simulink model "series_link_blance_leg"  (R2022b)
settings: Solver=ode45  StartTime=0.0  StopTime=14  MaxStep=0.2  RelTol=1e-3
values from neighbouring files (symbols this model uses):
  a11 = polyfit(leg,k11,2)    [series_get_k.m]
  a12 = polyfit(leg,k12,2)    [series_get_k.m]
  a13 = polyfit(leg,k13,1)    [series_get_k.m]
  a14 = polyfit(leg,k14,2)    [series_get_k.m]
  N = mp*diff(x + L*sin(theta),t,2)    [series_get_k1_length.m]
undefined symbols (not defined in the file or in its folder): X, Y, Z
libraries: sm_lib x74, nesl_utility x17, slpidlib x2, cstblocks x2, matrix_library x2
(part 3 of 3)

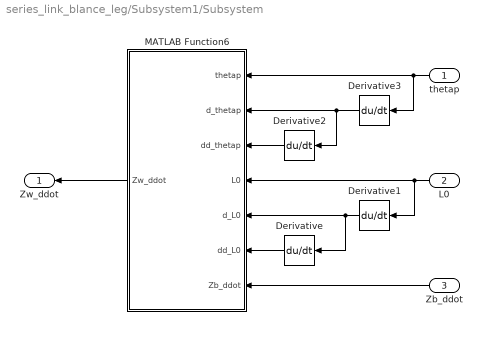
== system series_link_blance_leg/Subsystem1/Subsystem ==
  thetap : Inport
  L0 : Inport  Port=2
  Zb_ddot : Inport  Port=3
  Derivative{,1..3} (4 alike) : Derivative
  MATLAB Function6 : MATLAB Function  TreatAsAtomicUnit=on
  Zw_ddot : Outport
  wires:
  thetap/1 -> MATLAB Function6/1(thetap), Derivative3/1
  L0/1 -> Derivative1/1, MATLAB Function6/4(L0)
  Derivative1/1 -> Derivative/1, MATLAB Function6/5(d_L0)
  Derivative2/1 -> MATLAB Function6/3(dd_thetap)
  Derivative3/1 -> Derivative2/1, MATLAB Function6/2(d_thetap)
  Derivative/1 -> MATLAB Function6/6(dd_L0)
  Zb_ddot/1 -> MATLAB Function6/7(Zb_ddot)
  MATLAB Function6/1(Zw_ddot) -> Zw_ddot/1

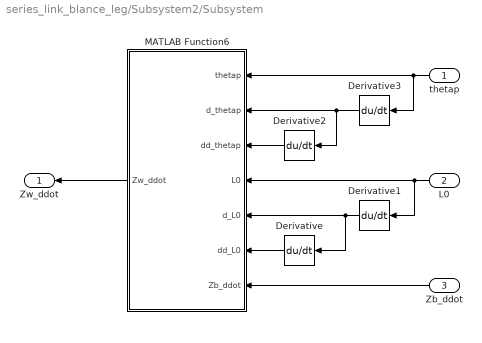
== system series_link_blance_leg/Subsystem2/Subsystem ==
  thetap : Inport
  L0 : Inport  Port=2
  Zb_ddot : Inport  Port=3
  Derivative{,1..3} (4 alike) : Derivative
  MATLAB Function6 : MATLAB Function  TreatAsAtomicUnit=on
  Zw_ddot : Outport
  wires:
  MATLAB Function6/1(Zw_ddot) -> Zw_ddot/1
  Zb_ddot/1 -> MATLAB Function6/7(Zb_ddot)
  Derivative/1 -> MATLAB Function6/6(dd_L0)
  Derivative3/1 -> MATLAB Function6/2(d_thetap), Derivative2/1
  Derivative2/1 -> MATLAB Function6/3(dd_thetap)
  Derivative1/1 -> MATLAB Function6/5(d_L0), Derivative/1
  L0/1 -> MATLAB Function6/4(L0), Derivative1/1
  thetap/1 -> Derivative3/1, MATLAB Function6/1(thetap)

== matlab function series_link_blance_leg/calc1/MATLAB Function6 ==
  data: k output; a input; length input
function k = get_K(a,length)
   k = polyval(a,length);  
end

== matlab function series_link_blance_leg/Subsystem1/Subsystem/MATLAB Function6 ==
  data: thetap input; Zw_ddot output; d_thetap input; dd_thetap input; L0 input; d_L0 input; dd_L0 input; Zb_ddot input
function Zw_ddot = Zw_ddot_calc(thetap,d_thetap,dd_thetap,L0,d_L0,dd_L0,Zb_ddot)

   Zw_ddot=Zb_ddot-dd_L0*cos(thetap)+2*d_L0*d_thetap*sin(thetap)+L0*dd_thetap*sin(thetap)+L0*(d_thetap^2)*cos(thetap);
end

== matlab function series_link_blance_leg/Subsystem1/MATLAB Function6 ==
  data: thetap input; zw_ddot input; F input; Fn output
function Fn = Fn_calc(thetap,zw_ddot,F)
    
  Mp=5.54; 
  Mw=1.18;
  g=9.8;
  Fn=F*cos(thetap)+Mp*g+Mw*zw_ddot;
end

== matlab function series_link_blance_leg/Subsystem2/MATLAB Function6 ==
  data: thetap input; zw_ddot input; F input; Fn output
function Fn = Fn_calc(thetap,zw_ddot,F)
    
  Mp=5.54; 
  Mw=1.18;
  g=9.8;
  Fn=F*cos(thetap)+Mp*g+Mw*zw_ddot;
end

== matlab function series_link_blance_leg/Subsystem2/Subsystem/MATLAB Function6 ==
  data: thetap input; Zw_ddot output; d_thetap input; dd_thetap input; L0 input; d_L0 input; dd_L0 input; Zb_ddot input
function Zw_ddot = Zw_ddot_calc(thetap,d_thetap,dd_thetap,L0,d_L0,dd_L0,Zb_ddot)

   Zw_ddot=Zb_ddot-dd_L0*cos(thetap)+2*d_L0*d_thetap*sin(thetap)+L0*dd_thetap*sin(thetap)+L0*(d_thetap^2)*cos(thetap);
end

== matlab function series_link_blance_leg/control1/MATLAB Function6 ==
  data: F0 input; T_joint output; theta1 input
function T_joint = VMC_calc(F0,theta1)
    l1 = 0.163; %%163.04mm
    l2 = 0.165; %%164.75mm
    l3 = 0.170; %%170.15mm
    l4 = 0.08;  %%79.5mm
    l23 = 0.04;  %%40.05mm

    J = l2*cos(theta1) + l1*cos(theta1 + acos((l2^2 - 2*cos(pi/4 + theta1)*l2*l4 - l3^2 + l4^2 + l23^2)/(2*l23*(l2^2 - 2*cos(pi/4 + theta1)*l2*l4 + l4^2)^(1/2))) + asin((l4*sin(theta1 + pi/4))/(l2^2 - 2*cos(pi/4 + theta1)*l2*l4 + l4^2)^(1/2)))*(((l4*cos(theta1 + pi/4))/(l2^2 - 2*cos(pi/4 + theta1)*l2*l4 + l4^2)^(1/2) - (l2*l4^2*sin(theta1 + pi/4)^2)/(l2^2 - 2*cos(pi/4 + theta1)*l2*l4 + l4^2)^(3/2))/(1 - (l4^2*sin(theta1 + pi/4)^2)/(l2^2 - 2*cos(pi/4 + theta1)*l2*l4 + l4^2))^(1/2) - ((l2*l4*sin(theta1 + pi/4))/(l23*(l2^2 - 2*cos(pi/4 + theta1)*l2*l4 + l4^2)^(1/2)) - (l2*l4*sin(theta1 + pi/4)*(l2^2 - 2*cos(pi/4 + theta1)*l2*l4 - l3^2 + l4^2 + l23^2))/(2*l23*(l2^2 - 2*cos(pi/4 + theta1)*l2*l4 + l4^2)^(3/2)))/(1 - (l2^2 - 2*cos(pi/4 + theta1)*l2*l4 - l3^2 + l4^2 + l23^2)^2/(4*l23^2*(l2^2 - 2*cos(pi/4 + theta1)*l2*l4 + l4^2)))^(1/2) + 1);
    T_joint = F0*J;

end

== matlab function series_link_blance_leg/control1/MATLAB Function7 ==
  data: L0 output; theta1 input
function L0 = L0(theta1)
    l1 = 0.163; %%163.04mm
    l2 = 0.165; %%164.75mm
    l3 = 0.170; %%170.15mm
    l4 = 0.08;  %%79.5mm
    l23 = 0.04;  %%40.05mm

    
    l5 = sqrt(l2^2 + l4^2 -2*l2*l4*cos(theta1 + pi/4));
    theta2 = asin(l4*sin(theta1 + pi/4)/l5);
    theta3 = acos((l23^2+l5^2-l3^2)/(2*l23*l5));
    theta4 =theta1 + theta2 +theta3;
    yc = l2*sin(theta1) + l1*sin(theta4);
    L0 = yc;

end

== matlab function series_link_blance_leg/calc/MATLAB Function6 ==
  data: k output; a input; length input
function k = get_K(a,length)
   k = polyval(a,length);  
end

== matlab function series_link_blance_leg/calc/MATLAB Function1 ==
  data: k output; a input; length input
function k = get_K(a,length)
   k = polyval(a,length);  
end

== matlab function series_link_blance_leg/calc/MATLAB Function2 ==
  data: k output; a input; length input
function k = get_K(a,length)
   k = polyval(a,length);  
end

== matlab function series_link_blance_leg/calc/MATLAB Function3 ==
  data: k output; a input; length input
function k = get_K(a,length)
   k = polyval(a,length);  
end

== matlab function series_link_blance_leg/calc1/MATLAB Function1 ==
  data: k output; a input; length input
function k = get_K(a,length)
   k = polyval(a,length);  
end

== matlab function series_link_blance_leg/calc1/MATLAB Function2 ==
  data: k output; a input; length input
function k = get_K(a,length)
   k = polyval(a,length);  
end

== matlab function series_link_blance_leg/control/MATLAB Function6 ==
  data: F0 input; T_joint output; theta1 input
function T_joint = VMC_calc(F0,theta1)
    l1 = 0.163; %%163.04mm
    l2 = 0.165; %%164.75mm
    l3 = 0.170; %%170.15mm
    l4 = 0.08;  %%79.5mm
    l23 = 0.04;  %%40.05mm

    J = l2*cos(theta1) + l1*cos(theta1 + acos((l2^2 - 2*cos(pi/4 + theta1)*l2*l4 - l3^2 + l4^2 + l23^2)/(2*l23*(l2^2 - 2*cos(pi/4 + theta1)*l2*l4 + l4^2)^(1/2))) + asin((l4*sin(theta1 + pi/4))/(l2^2 - 2*cos(pi/4 + theta1)*l2*l4 + l4^2)^(1/2)))*(((l4*cos(theta1 + pi/4))/(l2^2 - 2*cos(pi/4 + theta1)*l2*l4 + l4^2)^(1/2) - (l2*l4^2*sin(theta1 + pi/4)^2)/(l2^2 - 2*cos(pi/4 + theta1)*l2*l4 + l4^2)^(3/2))/(1 - (l4^2*sin(theta1 + pi/4)^2)/(l2^2 - 2*cos(pi/4 + theta1)*l2*l4 + l4^2))^(1/2) - ((l2*l4*sin(theta1 + pi/4))/(l23*(l2^2 - 2*cos(pi/4 + theta1)*l2*l4 + l4^2)^(1/2)) - (l2*l4*sin(theta1 + pi/4)*(l2^2 - 2*cos(pi/4 + theta1)*l2*l4 - l3^2 + l4^2 + l23^2))/(2*l23*(l2^2 - 2*cos(pi/4 + theta1)*l2*l4 + l4^2)^(3/2)))/(1 - (l2^2 - 2*cos(pi/4 + theta1)*l2*l4 - l3^2 + l4^2 + l23^2)^2/(4*l23^2*(l2^2 - 2*cos(pi/4 + theta1)*l2*l4 + l4^2)))^(1/2) + 1);
    T_joint = F0*J;

end

== matlab function series_link_blance_leg/control/MATLAB Function7 ==
  data: L0 output; theta1 input
function L0 = L0(theta1)
    l1 = 0.163; %%163.04mm
    l2 = 0.165; %%164.75mm
    l3 = 0.170; %%170.15mm
    l4 = 0.08;  %%79.5mm
    l23 = 0.04;  %%40.05mm

    
    l5 = sqrt(l2^2 + l4^2 -2*l2*l4*cos(theta1 + pi/4));
    theta2 = asin(l4*sin(theta1 + pi/4)/l5);
    theta3 = acos((l23^2+l5^2-l3^2)/(2*l23*l5));
    theta4 =theta1 + theta2 +theta3;
    yc = l2*sin(theta1) + l1*sin(theta4);
    L0 = yc;

end

== matlab function series_link_blance_leg/calc1/MATLAB Function3 ==
  data: k output; a input; length input
function k = get_K(a,length)
   k = polyval(a,length);  
end
